simulink model "expt_5_c"  (R2018b)
settings: Solver=VariableStepAuto  StartTime=0.0  StopTime=10e-3  RelTol=1e-3
libraries: commrandsrc3 x1
settings Model: Creator=sangh  LastModifiedBy=sangh

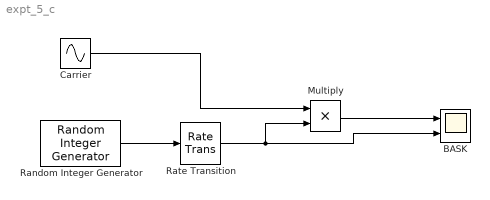
== system expt_5_c ==
  BASK : Scope  NumInputPorts=2
  Carrier : Sin  Amplitude=5  Frequency=20e3  SampleTime=2e-6
  Multiply : Product
  Random Integer Generator : commrandsrc3/Random Integer Generator  SetSize=2  SeedSource=Auto  Seed=0  SampleTime=0.001  SamplesPerFrame=1  OutputDataType=boolean  SimulateUsing=Interpreted execution
  Rate Transition : RateTransition  OutPortSampleTime=2e-6
  wires:
  Random Integer Generator/1 -> Rate Transition/1
  Rate Transition/1 -> BASK/2, Multiply/2
  Carrier/1 -> Multiply/1
  Multiply/1 -> BASK/1
